simulink subsystem "Observer_Front"  (R2023a)
settings: Solver=VariableStepAuto  StartTime=0.0  StopTime=10.0  RelTol=1e-3
undefined symbols (not defined in the file): A_front, b_front, C_out, observer_front, Ts
settings Model: Creator=morit  LastModifiedBy=morit

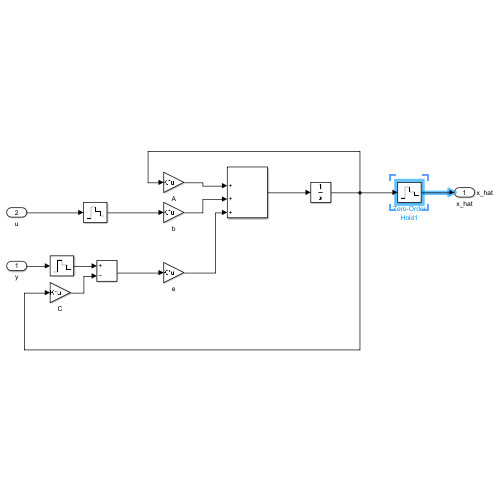
[thumbnail: Simulink's stored preview of the top-level diagram]
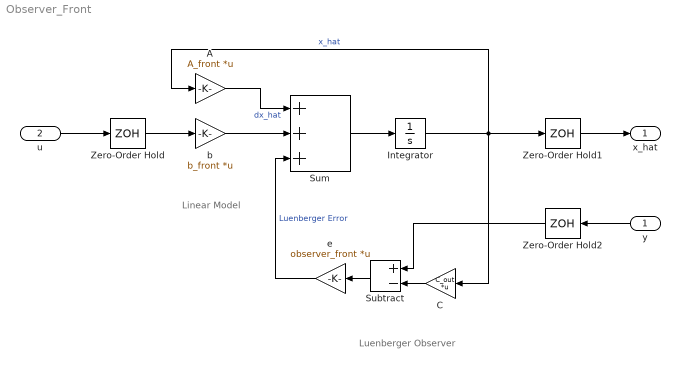
== system Observer_Front ==
  note: Linear Model
  note: Luenberger Observer
  y : Inport
  u : Inport  Port=2
  A : Gain  Gain=A_front  Multiplication=Matrix(K*u)
  C : Gain  Gain=C_out  Multiplication=Matrix(K*u)
  Integrator : Integrator
  Subtract : Sum  Inputs=+-
  Sum : Sum  Inputs=+++
  Zero-Order Hold : ZeroOrderHold  SampleTime=Ts
  Zero-Order Hold1 : ZeroOrderHold  SampleTime=Ts
  Zero-Order Hold2 : ZeroOrderHold  SampleTime=Ts
  b : Gain  Gain=b_front  Multiplication=Matrix(K*u)
  e : Gain  Gain=observer_front  Multiplication=Matrix(K*u)
  x_hat : Outport  SignalName=x_hat
  wires:
  Integrator/1 -> C/1, Zero-Order Hold1/1, A/1  "x_hat"
  Sum/1 -> Integrator/1
  A/1 -> Sum/1  "dx_hat"
  u/1 -> Zero-Order Hold/1
  b/1 -> Sum/2
  y/1 -> Zero-Order Hold2/1
  C/1 -> Subtract/2
  Subtract/1 -> e/1
  Zero-Order Hold/1 -> b/1
  Zero-Order Hold1/1 -> x_hat/1
  Zero-Order Hold2/1 -> Subtract/1
  e/1 -> Sum/3  "Luenberger Error"
